simulink model "Part1FullModel"  (R2017a)
settings: Solver=VariableStepAuto  StartTime=0.0  StopTime=500  RelTol=1e-3
values from neighbouring files (symbols this model uses):
  A = [-0.322, 0.052, 0.028, -1.12, 0.002 ... (first row only)    [InitialisePart1.m]
  a_phi_1 = 2.87    [InitialisePart1.m]    (also in init.m)
  a_phi_2 = -0.65    [InitialisePart1.m]    (also in init.m)
  B = [0; 0; 0; 0; -7.5]    [InitialisePart1.m]
  d = 1.5*deg2rad    (= 0.0261799387799)    [InitialisePart1.m]    (also in init.m)
  g = 9.81    [InitialisePart1.m]    (also in init.m = -9.81)
  k_d_phi = (2*zeta*omega_n-a_phi_1)/a_phi_2    [InitialisePart1.m]    (also in init.m)
  k_i_khi = (V_g/g)*(omega_x)^2    [InitialisePart1.m]    (also in init.m)
  k_i_phi = -1    [InitialisePart1.m]    (also in init.m = 1)
  k_p_khi = (V_g/g)*2*zeta_x*omega_x    [InitialisePart1.m]    (also in init.m)
  k_p_phi = delta_a_max/e_max*sign(a_phi_2)    [InitialisePart1.m]    (also in init.m)
  V_g = V_a    (= 161.111111111)    [InitialisePart1.m]    (also in init.m)
settings Model: Creator=martimos  LastModifiedBy=Ambjørn

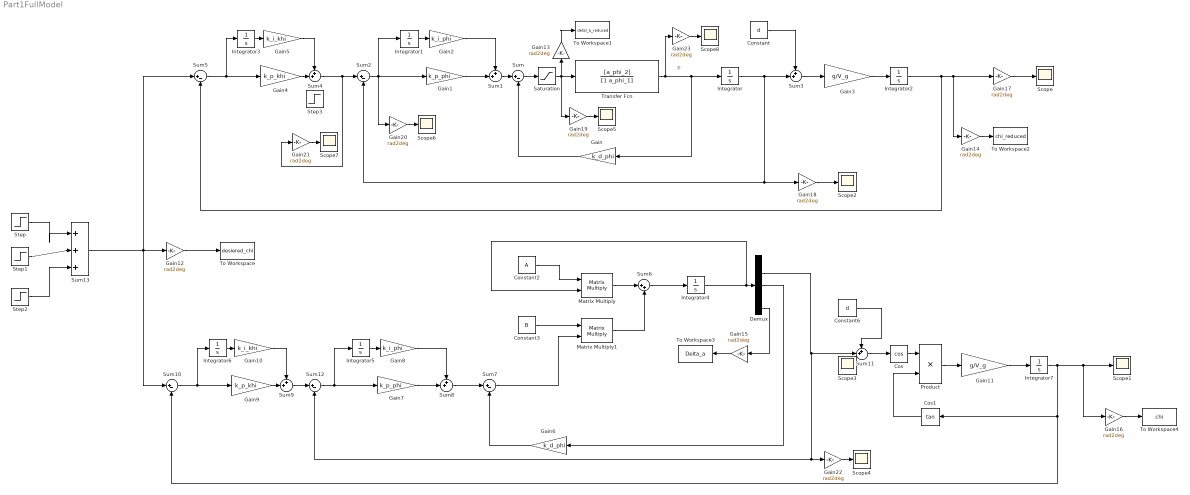
== system Part1FullModel ==
  note: p
  Constant : Constant  Value=d
  Constant2 : Constant  Value=A
  Constant3 : Constant  Value=B
  Constant6 : Constant  Value=d
  Cos : Trigonometry  Operator=cos
  Cos1 : Trigonometry  Operator=tan
  Demux : Demux  Outputs=5
  Gain : Gain  Gain=k_d_phi
  Gain1 : Gain  Gain=k_p_phi
  Gain10 : Gain  Gain=k_i_khi
  Gain11 : Gain  Gain=g/V_g
  Gain{12..23} (12 alike) : Gain  Gain=rad2deg
  Gain2 : Gain  Gain=k_i_phi
  Gain3 : Gain  Gain=g/V_g
  Gain4 : Gain  Gain=k_p_khi
  Gain5 : Gain  Gain=k_i_khi
  Gain6 : Gain  Gain=k_d_phi
  Gain7 : Gain  Gain=k_p_phi
  Gain8 : Gain  Gain=k_i_phi
  Gain9 : Gain  Gain=k_p_khi
  Integrator{,1..7} (8 alike) : Integrator
  Matrix Multiply : Product  Multiplication=Matrix(*)
  Matrix Multiply1 : Product  Multiplication=Matrix(*)
  Product : Product
  Saturation : Saturate  UpperLimit=30*deg2rad  LowerLimit=-30*deg2rad
  Scope{,1..8} (9 alike) : Scope
  Step : Step  Time=5  After=2*deg2rad  SampleTime=0
  Step1 : Step  Time=15  After=-0*deg2rad  SampleTime=0
  Step2 : Step  Time=25  After=-0*deg2rad  SampleTime=0
  Step3 : Step  Time=5  After=15*deg2rad  SampleTime=0
  Sum{,2,5,7,10,12} (6 alike) : Sum  Inputs=|+-
  Sum{1,3..4,8..9,11} (6 alike) : Sum  Inputs=++|
  Sum13 : Sum  Inputs=|+++
  Sum6 : Sum  Inputs=|++
  To Workspace : ToWorkspace  VariableName=desiered_chi  SaveFormat=Timeseries  SampleTime=-1
  To Workspace1 : ToWorkspace  VariableName=detal_a_reduced  SaveFormat=Timeseries  SampleTime=-1
  To Workspace2 : ToWorkspace  VariableName=chi_reduced  SaveFormat=Timeseries  SampleTime=-1
  To Workspace3 : ToWorkspace  VariableName=Delta_a  SaveFormat=Timeseries  SampleTime=-1
  To Workspace4 : ToWorkspace  VariableName=chi  SaveFormat=Timeseries  SampleTime=-1
  Transfer Fcn : TransferFcn  Numerator=[a_phi_2]  Denominator=[1 a_phi_1]
  wires:
  Transfer Fcn/1 -> Gain23/1, Gain/1, Integrator/1
  Sum/1 -> Saturation/1
  Gain/1 -> Sum/2
  Sum1/1 -> Sum/1
  Gain1/1 -> Sum1/2
  Gain2/1 -> Sum1/1
  Sum2/1 -> Gain20/1, Integrator1/1, Gain1/1
  Integrator1/1 -> Gain2/1
  Integrator/1 -> Sum3/2, Sum2/2, Gain18/1
  Sum3/1 -> Gain3/1
  Constant/1 -> Sum3/1
  Gain3/1 -> Integrator2/1
  Integrator2/1 -> Sum5/2, Gain14/1, Gain17/1
  Gain4/1 -> Sum4/2
  Gain5/1 -> Sum4/1
  Sum5/1 -> Integrator3/1, Gain4/1
  Integrator3/1 -> Gain5/1
  Sum6/1 -> Integrator4/1
  Constant2/1 -> Matrix Multiply/1
  Matrix Multiply/1 -> Sum6/1
  Matrix Multiply1/1 -> Sum6/2
  Constant3/1 -> Matrix Multiply1/1
  Integrator4/1 -> Demux/1, Matrix Multiply/2
  Gain7/1 -> Sum8/2
  Sum8/1 -> Sum7/1
  Integrator5/1 -> Gain8/1
  Gain8/1 -> Sum8/1
  Gain6/1 -> Sum7/2
  Sum10/1 -> Integrator6/1, Gain9/1
  Gain10/1 -> Sum9/1
  Gain9/1 -> Sum9/2
  Sum13/1 -> Gain12/1, Sum5/1, Sum10/1
  Constant6/1 -> Sum11/1
  Demux/2 -> Sum12/2, Gain22/1, Sum11/2
  Integrator7/1 -> Gain16/1, Scope1/1, Cos1/1, Sum10/2
  Sum11/1 -> Cos/1
  Gain11/1 -> Integrator7/1
  Demux/3 -> Gain6/1
  Integrator6/1 -> Gain10/1
  Product/1 -> Gain11/1
  Cos/1 -> Product/1
  Cos1/1 -> Product/2
  Sum7/1 -> Matrix Multiply1/2
  Sum9/1 -> Sum12/1
  Sum12/1 -> Integrator5/1, Gain7/1
  Step/1 -> Sum13/1
  Step1/1 -> Sum13/2
  Step2/1 -> Sum13/3
  Gain12/1 -> To Workspace/1
  Gain13/1 -> To Workspace1/1
  Gain14/1 -> To Workspace2/1
  Demux/5 -> Gain15/1
  Gain15/1 -> To Workspace3/1
  Gain16/1 -> To Workspace4/1
  Gain17/1 -> Scope/1
  Gain18/1 -> Scope2/1
  Saturation/1 -> Gain19/1, Gain13/1, Transfer Fcn/1
  Gain19/1 -> Scope5/1
  Gain20/1 -> Scope6/1
  Gain21/1 -> Scope7/1
  Gain22/1 -> Scope4/1
  Gain23/1 -> Scope8/1
  Sum4/1 -> Gain21/1, Sum2/1
